simulink model "sampleModel1776"  (R2023a)
settings: Solver=VariableStepAuto  StartTime=0.0  StopTime=10.0  RelTol=1e-3
libraries: hdlsllib x3
settings Model: Creator=user1  LastModifiedBy=user1

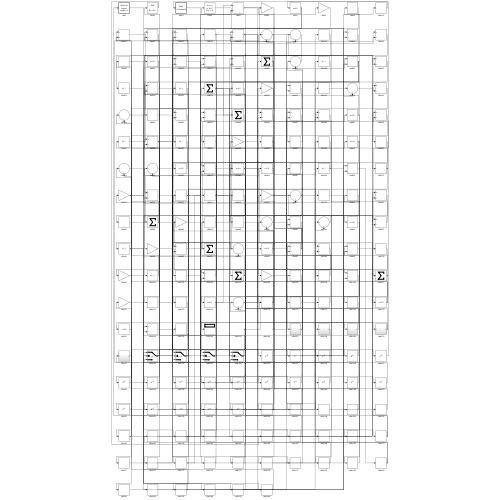
[thumbnail: Simulink's stored preview of the top-level diagram]
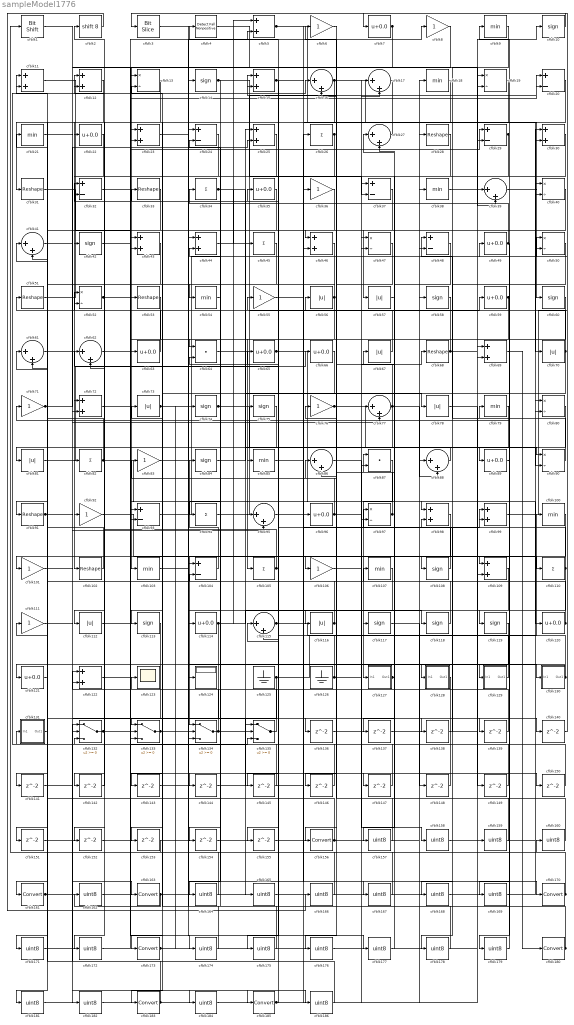
== system sampleModel1776 ==
  cfblk1 : hdlsllib/Logic and Bit Operations/Bit Shift  mode=Shift Left Logical  N=0
  cfblk{10,14,42,58,60,74..75,84,108,113,117..119} (13 alike) : Signum
  cfblk{9,18,21,38,54,79,85,100,103,107} (10 alike) : MinMax
  cfblk{6,8,36,55,71,76,83,92,101,106,111} (11 alike) : Gain
  cfblk{28,31,33,51,53,68,91,102} (8 alike) : Reshape
  cfblk{20,24,29,32,37,48,93,104} (8 alike) : Sum  Inputs=+-
  cfblk{26,34,45,82,94,105,110} (7 alike) : Sum  Inputs=+
  cfblk{5,11..12,15,23,25,30,43..44,46,69,72,98..99,109,122} (16 alike) : Sum
  cfblk{56..57,67,70,73,78,81,112,116} (9 alike) : Abs  SaturateOnIntegerOverflow=off
  cfblk{7,22,35,49,59,63,65..66,89,96,114,120..121} (13 alike) : Bias  Bias=0.0  SaturateOnIntegerOverflow=off
  cfblk{16..17,27,39,41,61..62,77,86,88,95,115} (12 alike) : Sum  Inputs=|++
  cfblk123 : Scope
  cfblk124 : Display
  cfblk125 : Ground
  cfblk126 : Ground
  cfblk127 : Subsystem
      settings: LibrarySourceBlock=|
      | hdlsllib/Ports &
      | Subsystems/Subsystem
  cfblk128 : Subsystem
      settings: LibrarySourceBlock=|
      | hdlsllib/Ports &
      | Subsystems/Subsystem
  cfblk129 : Subsystem
      settings: LibrarySourceBlock=|
      | hdlsllib/Ports &
      | Subsystems/Subsystem
  cfblk{13,19,40,47,50,52,80,90,97} (9 alike) : Product  Inputs=*/  RndMeth=Zero  SaturateOnIntegerOverflow=on
  cfblk130 : Subsystem
      settings: LibrarySourceBlock=|
      | hdlsllib/Ports &
      | Subsystems/Subsystem
  cfblk131 : Subsystem
      settings: LibrarySourceBlock=|
      | hdlsllib/Ports &
      | Subsystems/Subsystem
  cfblk{132..135} (4 alike) : Switch  SaturateOnIntegerOverflow=off  InputSameDT=off
  cfblk{136..155} (20 alike) : Delay  SampleTime=1
  cfblk{156,161,163,170,173,180,183,185} (8 alike) : DataTypeConversion  SaturateOnIntegerOverflow=off  RndMeth=Floor
  cfblk{157..160,162,164..169,171..172,174..179,181..182,184,186} (23 alike) : DataTypeConversion  OutDataTypeStr=uint8  SaturateOnIntegerOverflow=off  RndMeth=Floor
  cfblk2 : ArithShift  BitShiftNumber=8
  cfblk3 : hdlsllib/Logic and Bit Operations/Bit Slice  lidx=7  ridx=0
  cfblk4 : hdlsllib/Logic and Bit Operations/Detect Fall Nonpositive  vinit=0  OutDataTypeStr=boolean
  cfblk64 : DotProduct  OutDataTypeStr=Inherit: Inherit via internal rule
  cfblk87 : DotProduct  OutDataTypeStr=Inherit: Inherit via internal rule
  wires:
  cfblk134/1 -> cfblk123/1, cfblk138/1
  cfblk59/1 -> cfblk71/1, cfblk135/2
  cfblk92/1 -> cfblk109/1
  cfblk75/1 -> cfblk103/1
  cfblk5/1 -> cfblk60/1, cfblk30/2
  cfblk58/1 -> cfblk105/1
  cfblk98/1 -> cfblk134/1
  cfblk63/1 -> cfblk51/1
  cfblk88/1 -> cfblk81/1
  cfblk99/1 -> cfblk3/1
  cfblk13/1 -> cfblk31/1
  cfblk71/1 -> cfblk25/2, cfblk186/1
  cfblk64/1 -> cfblk20/1
  cfblk128/1(Out1) -> cfblk12/1
  cfblk53/1 -> cfblk93/1
  cfblk23/1 -> cfblk170/1
  cfblk69/1 -> cfblk180/1
  cfblk8/1 -> cfblk63/1
  cfblk10/1 -> cfblk7/1
  cfblk94/1 -> cfblk56/1
  cfblk115/1 -> cfblk100/1, cfblk59/1
  cfblk22/1 -> cfblk102/1
  cfblk26/1 -> cfblk112/1, cfblk54/1
  cfblk89/1 -> cfblk119/1
  cfblk129/1(Out1) -> cfblk4/1
  cfblk11/1 -> cfblk16/1
  cfblk105/1 -> cfblk2/1, cfblk155/1
  cfblk6/1 -> cfblk156/1
  cfblk76/1 -> cfblk89/1, cfblk17/2, cfblk49/1
  cfblk116/1 -> cfblk114/1, cfblk32/1
  cfblk111/1 -> cfblk163/1
  cfblk51/1 -> cfblk15/1
  cfblk36/1 -> cfblk183/1
  cfblk28/1 -> cfblk85/1
  cfblk40/1 -> cfblk57/1
  cfblk114/1 -> cfblk75/1, cfblk118/1, cfblk171/1
  cfblk18/1 -> cfblk161/1
  cfblk74/1 -> cfblk90/1, cfblk88/2, cfblk5/1
  cfblk87/1 -> cfblk127/1(In1)
  cfblk52/1 -> cfblk97/2, cfblk139/1
  cfblk96/1 -> cfblk47/1, cfblk83/1
  cfblk66/1 -> cfblk113/1
  cfblk15/1 -> cfblk96/1, cfblk145/1, cfblk167/1
  cfblk65/1 -> cfblk120/1, cfblk130/1(In1)
  cfblk93/1 -> cfblk28/1
  cfblk17/1 -> cfblk43/1
  cfblk55/1 -> cfblk50/1
  cfblk30/1 -> cfblk117/1
  cfblk39/1 -> cfblk40/2
  cfblk104/1 -> cfblk84/1
  cfblk14/1 -> cfblk37/2, cfblk104/1
  cfblk3/1 -> cfblk134/2
  cfblk127/1(Out1) -> cfblk67/1, cfblk97/1
  cfblk38/1 -> cfblk39/1
  cfblk24/1 -> cfblk173/1
  cfblk73/1 -> cfblk5/2, cfblk147/1
  cfblk45/1 -> cfblk124/1
  cfblk68/1 -> cfblk10/1, cfblk64/1
  cfblk97/1 -> cfblk76/1, cfblk15/2
  cfblk12/1 -> cfblk92/1
  cfblk34/1 -> cfblk78/1, cfblk45/1, cfblk150/1
  cfblk1/1 -> cfblk19/2
  cfblk25/1 -> cfblk134/3
  cfblk35/1 -> cfblk91/1
  cfblk70/1 -> cfblk33/1, cfblk143/1
  cfblk81/1 -> cfblk66/1
  cfblk20/1 -> cfblk42/1
  cfblk91/1 -> cfblk133/1, cfblk95/2
  cfblk135/1 -> cfblk52/1
  cfblk77/1 -> cfblk122/2, cfblk90/2, cfblk16/2
  cfblk132/1 -> cfblk12/2, cfblk20/2, cfblk135/3
  cfblk83/1 -> cfblk129/1(In1)
  cfblk37/1 -> cfblk115/2
  cfblk50/1 -> cfblk108/1
  cfblk118/1 -> cfblk11/1
  cfblk122/1 -> cfblk29/1
  cfblk41/1 -> cfblk77/2
  cfblk56/1 -> cfblk53/1, cfblk93/2, cfblk153/1
  cfblk120/1 -> cfblk99/1, cfblk104/2
  cfblk19/1 -> cfblk82/1
  cfblk61/1 -> cfblk72/1
  cfblk110/1 -> cfblk87/1, cfblk175/1
  cfblk106/1 -> cfblk47/2
  cfblk130/1(Out1) -> cfblk128/1(In1), cfblk64/2
  cfblk16/1 -> cfblk70/1, cfblk133/2
  cfblk82/1 -> cfblk41/2, cfblk95/1
  cfblk125/1 -> cfblk87/2, cfblk172/1
  cfblk7/1 -> cfblk72/2, cfblk133/3
  cfblk31/1 -> cfblk43/2
  cfblk84/1 -> cfblk25/1
  cfblk67/1 -> cfblk11/2
  cfblk108/1 -> cfblk62/1
  cfblk43/1 -> cfblk121/1
  cfblk49/1 -> cfblk34/1, cfblk179/1
  cfblk126/1 -> cfblk68/1, cfblk32/2
  cfblk21/1 -> cfblk185/1
  cfblk47/1 -> cfblk116/1
  cfblk4/1 -> cfblk39/2
  cfblk95/1 -> cfblk99/2
  cfblk102/1 -> cfblk61/2
  cfblk90/1 -> cfblk48/1
  cfblk42/1 -> cfblk98/1
  cfblk29/1 -> cfblk46/1, cfblk94/1, cfblk106/1
  cfblk57/1 -> cfblk27/2
  cfblk62/1 -> cfblk8/1
  cfblk100/1 -> cfblk101/1
  cfblk133/1 -> cfblk13/2, cfblk140/1
  cfblk27/1 -> cfblk22/1
  cfblk85/1 -> cfblk110/1
  cfblk72/1 -> cfblk136/1
  cfblk136/1 -> cfblk29/2
  cfblk109/1 -> cfblk137/1
  cfblk137/1 -> cfblk19/1
  cfblk138/1 -> cfblk98/2
  cfblk139/1 -> cfblk122/1
  cfblk140/1 -> cfblk50/2
  cfblk121/1 -> cfblk141/1
  cfblk33/1 -> cfblk142/1
  cfblk142/1 -> cfblk62/2
  cfblk143/1 -> cfblk135/1
  cfblk32/1 -> cfblk144/1
  cfblk144/1 -> cfblk46/2
  cfblk145/1 -> cfblk132/1
  cfblk80/1 -> cfblk146/1
  cfblk146/1 -> cfblk52/2
  cfblk147/1 -> cfblk115/1
  cfblk117/1 -> cfblk148/1
  cfblk148/1 -> cfblk41/1
  cfblk78/1 -> cfblk149/1
  cfblk149/1 -> cfblk37/1
  cfblk150/1 -> cfblk132/3
  cfblk131/1(Out1) -> cfblk151/1
  cfblk151/1 -> cfblk77/1
  cfblk113/1 -> cfblk152/1
  cfblk152/1 -> cfblk88/1
  cfblk153/1 -> cfblk1/1
  cfblk54/1 -> cfblk154/1
  cfblk154/1 -> cfblk26/1
  cfblk155/1 -> cfblk58/1
  cfblk156/1 -> cfblk131/1(In1), cfblk13/1
  cfblk48/1 -> cfblk157/1
  cfblk157/1 -> cfblk6/1
  cfblk86/1 -> cfblk158/1
  cfblk158/1 -> cfblk40/1
  cfblk159/1 -> cfblk86/1
  cfblk160/1 -> cfblk86/2
  cfblk161/1 -> cfblk14/1, cfblk61/1
  cfblk162/1 -> cfblk18/1
  cfblk163/1 -> cfblk162/1, cfblk30/1
  cfblk46/1 -> cfblk164/1
  cfblk164/1 -> cfblk111/1
  cfblk44/1 -> cfblk165/1
  cfblk165/1 -> cfblk80/1
  cfblk2/1 -> cfblk166/1
  cfblk166/1 -> cfblk44/1
  cfblk167/1 -> cfblk44/2
  cfblk9/1 -> cfblk168/1
  cfblk168/1 -> cfblk80/2
  cfblk60/1 -> cfblk169/1
  cfblk169/1 -> cfblk9/1
  cfblk170/1 -> cfblk160/1, cfblk35/1
  cfblk171/1 -> cfblk23/1
  cfblk172/1 -> cfblk23/2
  cfblk173/1 -> cfblk159/1, cfblk74/1
  cfblk112/1 -> cfblk174/1
  cfblk174/1 -> cfblk24/1
  cfblk175/1 -> cfblk24/2
  cfblk107/1 -> cfblk176/1
  cfblk176/1 -> cfblk38/1
  cfblk103/1 -> cfblk177/1
  cfblk177/1 -> cfblk107/1
  cfblk79/1 -> cfblk178/1
  cfblk178/1 -> cfblk27/1
  cfblk179/1 -> cfblk79/1
  cfblk180/1 -> cfblk73/1, cfblk55/1
  cfblk119/1 -> cfblk181/1
  cfblk181/1 -> cfblk69/1
  cfblk141/1 -> cfblk182/1
  cfblk182/1 -> cfblk69/2
  cfblk183/1 -> cfblk132/2, cfblk109/2
  cfblk101/1 -> cfblk184/1
  cfblk184/1 -> cfblk36/1
  cfblk185/1 -> cfblk65/1, cfblk48/2, cfblk17/1
  cfblk186/1 -> cfblk21/1

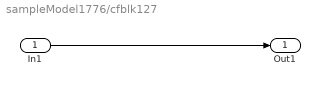
== system sampleModel1776/cfblk127 ==
  In1 : Inport
  Out1 : Outport
  wires:
  In1/1 -> Out1/1

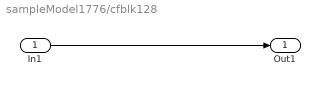
== system sampleModel1776/cfblk128 ==
  In1 : Inport
  Out1 : Outport
  wires:
  In1/1 -> Out1/1

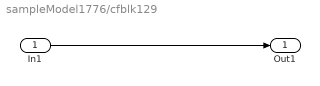
== system sampleModel1776/cfblk129 ==
  In1 : Inport
  Out1 : Outport
  wires:
  In1/1 -> Out1/1

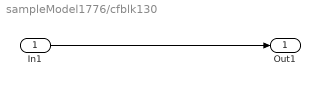
== system sampleModel1776/cfblk130 ==
  In1 : Inport
  Out1 : Outport
  wires:
  In1/1 -> Out1/1

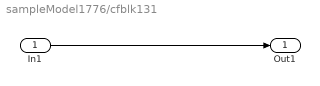
== system sampleModel1776/cfblk131 ==
  In1 : Inport
  Out1 : Outport
  wires:
  In1/1 -> Out1/1
